simulink model "Longitudinal_Guide_130"  (Simulink 7.2)
settings: Solver=ode45  StartTime=0.0  StopTime=10.0  RelTol=1e-3
undefined symbols (not defined in the file or in its folder): DiscIntNeverNeededParam
libraries: simulink x1
settings Model: Creator=arnaud  LastModifiedBy=arnaud

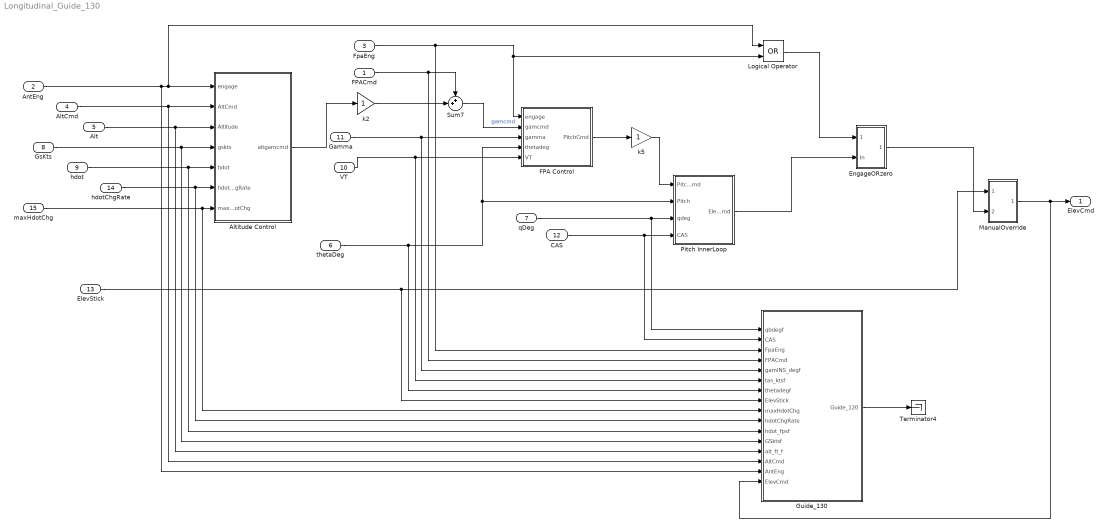
== system Longitudinal_Guide_130 ==
  FPACmd : Inport  DataType=double  OutDataTypeStr=double
  AntEng : Inport  Port=2  DataType=boolean  OutDataTypeStr=boolean
  FpaEng : Inport  Port=3  DataType=boolean  OutDataTypeStr=boolean
  AltCmd : Inport  Port=4  DataType=double  OutDataTypeStr=double
  Alt : Inport  Port=5  DataType=double  OutDataTypeStr=double
  thetaDeg : Inport  Port=6  DataType=double  OutDataTypeStr=double
  qDeg : Inport  Port=7  DataType=double  OutDataTypeStr=double
  GsKts : Inport  Port=8  DataType=double  OutDataTypeStr=double
  hdot : Inport  Port=9  DataType=double  OutDataTypeStr=double
  VT : Inport  Port=10  DataType=double  OutDataTypeStr=double
  Gamma : Inport  Port=11  DataType=double  OutDataTypeStr=double
  CAS : Inport  Port=12  DataType=double  OutDataTypeStr=double
  ElevStick : Inport  Port=13  DataType=double  OutDataTypeStr=double
  hdotChgRate : Inport  Port=14  DataType=double  OutDataTypeStr=double
  maxHdotChg : Inport  Port=15  DataType=double  OutDataTypeStr=double
  Altitude Control : Subsystem  RequirementInfo={'other' '..\..\tcm_requirements.docx' '@Simulink_requirement_item_14' 'true' 'Altitude Control' '' }  TreatAsAtomicUnit=on
  EngageORzero : Subsystem
  FPA Control : Subsystem  RequirementInfo={'other' '..\..\tcm_requirements.docx' '@Simulink_requirement_item_15' 'true' 'FPA Control' '' }  TreatAsAtomicUnit=on
  Guide_130 : Subsystem  TreatAsAtomicUnit=on  mask(Observer){AnnotationType=ensures, ObserverType=ellipsoid}
      mask prompts: AnnotationType "Type of annotation (pre/post...)"; ObserverType "Observer type"
      mask help:
      | Set an observer for the system.
      | The annotation type parameter sets the type of observer:
      | - requires : pre-condition
      | - ensures : post-condition
      | - assert : an assertion
      | - observer : the observer computes a special type of properties
      mask StyleString: popup(ensures|requires|assert|observer),edit
      mask CallbackString:
      | paramStr = get_param(gcb, 'MaskValues');
      | 
      | if strcmp(paramStr{1}(1),'o')
      |     set_param(gcb,'MaskVisibilities',{'on';'on'});
      |     paramStr{2} = 'ellipsoid';
      |     set_param(gcb,'MaskValues',paramStr);
      | else
      |     set_param(gcb,'MaskVisibilities',{'on';'off'});
      | end|paramStr = get_param(gcb, 'MaskValues');
      | 
      | if strcmp(paramStr{1}(1),'observer')
      |     set_param(gcb,'MaskVisibilities',{'on';'on'});
      |     paramStr{2} = 'ellipsoid';
      |     set_param(gcb,'MaskValues',paramStr);
      | else
      |     set_param(gcb,'MaskVisibilities',{'on';'off'});
      | end
      mask Display:
      | color('red');
      | text(0.5, 0.5, 'Observer Block', 'horizontalAlignment', 'center');
  Logical Operator : Logic  Operator=OR  AllPortsSameDT=off  OutDataTypeMode=boolean  OutDataTypeStr=boolean
  ManualOverride : Subsystem
  Pitch InnerLoop : Subsystem  RequirementInfo={'other' '..\..\tcm_requirements.docx' '@Simulink_requirement_item_17' 'true' 'Pitch InnerLoop' '' }  TreatAsAtomicUnit=on
  Sum7 : Sum  RequirementInfo={} %GIDa_92495686_3877_4412_b19f_22e099e095ee  Inputs=++|
  Terminator4 : Terminator
  k2 : Gain  RequirementInfo={} %GIDa_7e514706_5da4_4f1f_bf6c_0050dd9ce76d
  k5 : Gain  RequirementInfo={} %GIDa_b8b0ba7d_7fd3_4b03_b740_56530c3187c8
  ElevCmd : Outport
  wires:
  k2/1 -> Sum7/2
  Alt/1 -> Altitude Control/3(Altitude), Guide_130/13(alt_ft_f)
  thetaDeg/1 -> FPA Control/4(thetadeg), Pitch InnerLoop/2(Pitch), Guide_130/7(thetadegf)
  Gamma/1 -> FPA Control/3(gamma), Guide_130/5(gamINS_degf)
  AltCmd/1 -> Altitude Control/2(AltCmd), Guide_130/14(AltCmd)
  ManualOverride/1(Out) -> ElevCmd/1, Guide_130/16(ElevCmd)
  Altitude Control/1(altgamcmd) -> k2/1
  FPA Control/1(PitchCmd) -> k5/1
  hdot/1 -> Altitude Control/5(hdot), Guide_130/11(hdot_fpsf)
  Sum7/1 -> FPA Control/2(gamcmd)  "gamcmd"
  qDeg/1 -> Pitch InnerLoop/3(qdeg), Guide_130/1(qbdegf)
  GsKts/1 -> Altitude Control/4(gskts), Guide_130/12(GSktsf)
  VT/1 -> FPA Control/5(VT), Guide_130/6(tas_ktsf)
  FPACmd/1 -> Sum7/1, Guide_130/4(FPACmd)
  k5/1 -> Pitch InnerLoop/1(PitchCmd)
  FpaEng/1 -> Logical Operator/2, FPA Control/1(engage), Guide_130/3(FpaEng)
  CAS/1 -> Pitch InnerLoop/4(CAS), Guide_130/2(CAS)
  AntEng/1 -> Logical Operator/1, Altitude Control/1(engage), Guide_130/15(AntEng)
  ElevStick/1 -> ManualOverride/1(Man), Guide_130/8(ElevStick)
  Pitch InnerLoop/1(ElevCmd) -> EngageORzero/2(In)
  EngageORzero/1(Out) -> ManualOverride/2(Auto)
  Logical Operator/1 -> EngageORzero/1(Engage)
  maxHdotChg/1 -> Altitude Control/7(maxHdotChg), Guide_130/9(maxHdotChg)
  hdotChgRate/1 -> Altitude Control/6(hdotChgRate), Guide_130/10(hdotChgRate)
  Guide_130/1(Guide_120) -> Terminator4/1

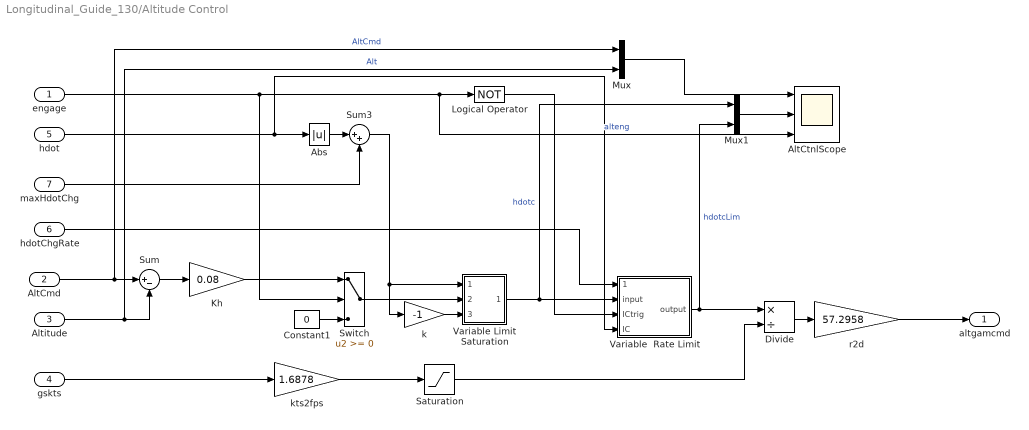
== system Longitudinal_Guide_130/Altitude Control ==
  engage : Inport  RequirementInfo={} %GIDa_92edc9e2_4cfd_4b16_8fee_8b94964575da
  AltCmd : Inport  RequirementInfo={} %GIDa_edbc7e5c_23e1_4d8f_98c5_e2d77895a510  Port=2
  Altitude : Inport  RequirementInfo={} %GIDa_01b40abf_ece8_4194_aeed_7639b2f9d320  Port=3
  gskts : Inport  RequirementInfo={} %GIDa_49aaf918_ec6b_4cc9_bdad_efb02f39ea3b  Port=4
  hdot : Inport  RequirementInfo={} %GIDa_f8353919_6ca2_40ed_9884_9c34b61b1365  Port=5
  hdotChgRate : Inport  Port=6
  maxHdotChg : Inport  Port=7
  Abs : Abs  RequirementInfo={} %GIDa_1391aa7c_5846_4be5_914e_111d8f2c4215  SaturateOnIntegerOverflow=on
  AltCtnlScope : Scope  NumInputPorts=3
      settings: RequirementInfo={} %GIDa_baad481c_a27b_41ac_bf32_d6e1a7f2cfe1  TimeRange=30  YMin=10000~-5~0  YMax=10200~15~1  SaveName=ScopeData3
  Constant1 : Constant  RequirementInfo={} %GIDa_566c4b52_316f_4d36_82bb_fb65e53f78d2  Value=0
  Divide : Product  RequirementInfo={} %GIDa_b9d1a3fe_7e00_46b2_9426_cf952dcaf391  Inputs=*/
  Kh : Gain  RequirementInfo={} %GIDa_de6b2d53_b3f4_42e2_83e9_439be9ccc299  Gain=0.08
  Logical Operator : Logic  RequirementInfo={} %GIDa_921e6188_0ac2_4a9c_befc_5c7a6835e9e6  Operator=NOT
  Mux : Mux  RequirementInfo={} %GIDa_68aa779e_2c07_4c3b_9ca1_0ecb3161e49a  Inputs=2
  Mux1 : Mux  RequirementInfo={} %GIDa_0a0909f8_d09a_4568_9828_3f29982a74b3  Inputs=2
  Saturation : Saturate  RequirementInfo={} %GIDa_77166b67_e163_40e1_b7e4_7e7410a56d29  UpperLimit=1000  LowerLimit=0.0001
  Sum : Sum  RequirementInfo={} %GIDa_d94a0856_9d8d_4fca_8b77_5f1cf21c0c3a  Inputs=|+-
  Sum3 : Sum  RequirementInfo={} %GIDa_3ee7802b_411f_4586_886f_8bdef6cfccb9  Inputs=|++  SaturateOnIntegerOverflow=on  InputSameDT=on  OutDataTypeStr=Inherit: Same as first input
  Switch : Switch  RequirementInfo={} %GIDa_64af29d5_be60_4de8_bcf5_833ab8e70f35
  Variable  Rate Limit : Subsystem  RequirementInfo={} %GIDa_7d0e1926_4469_4591_916e_2bb88ddee008  TreatAsAtomicUnit=on
  Variable Limit Saturation : Subsystem  RequirementInfo={} %GIDa_0b931211_59c1_4508_94b8_12d4cca2cb6b  TreatAsAtomicUnit=on
  k : Gain  RequirementInfo={} %GIDa_65a0c0b6_6e9b_4a97_b326_1d79079cc625  Gain=-1
  kts2fps : Gain  RequirementInfo={} %GIDa_a49848e7_9841_44de_8ec7_08f1ed28d1e0  Gain=1.6878
  r2d : Gain  RequirementInfo={} %GIDa_934ba914_aaac_471d_9b5e_a120031a3853  Gain=57.2958
  altgamcmd : Outport  RequirementInfo={} %GIDa_3c331913_004d_4e8f_a0a1_b052c80c7670
  wires:
  Sum/1 -> Kh/1
  AltCmd/1 -> Sum/1, Mux/1  "AltCmd"
  Altitude/1 -> Sum/2, Mux/2  "Alt"
  hdot/1 -> Abs/1, Variable  Rate Limit/4(IC)
  Abs/1 -> Sum3/1
  maxHdotChg/1 -> Sum3/2
  k/1 -> Variable Limit Saturation/3(Lo_lim)
  Sum3/1 -> k/1, Variable Limit Saturation/1(up_lim)
  engage/1 -> Switch/2, Logical Operator/1, AltCtnlScope/3  "alteng"
  gskts/1 -> kts2fps/1
  Divide/1 -> r2d/1
  r2d/1 -> altgamcmd/1
  Logical Operator/1 -> Variable  Rate Limit/3(ICtrig)
  Variable Limit Saturation/1(Out1) -> Variable  Rate Limit/2(input), Mux1/1  "hdotc"
  hdotChgRate/1 -> Variable  Rate Limit/1(ratelim)
  Variable  Rate Limit/1(output) -> Divide/1, Mux1/2  "hdotcLim"
  kts2fps/1 -> Saturation/1
  Saturation/1 -> Divide/2
  Switch/1 -> Variable Limit Saturation/2(SigIn)
  Kh/1 -> Switch/1
  Constant1/1 -> Switch/3
  Mux/1 -> AltCtnlScope/1
  Mux1/1 -> AltCtnlScope/2

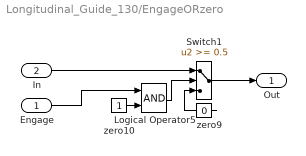
== system Longitudinal_Guide_130/EngageORzero ==
  Engage : Inport
  In : Inport  Port=2
  Logical Operator5 : Logic  RequirementInfo={} %GIDa_2faaa958_fdd5_4161_8224_87bc655595ec  AllPortsSameDT=off  OutDataTypeMode=boolean  OutDataTypeStr=boolean
  Switch1 : Switch  RequirementInfo={} %GIDa_cd8505b1_f38c_41a3_a83c_5e083797b181  Threshold=0.5
  zero10 : Constant  RequirementInfo={} %GIDa_596a5899_ba53_4c37_8272_7211e27ddf24
  zero9 : Constant  RequirementInfo={} %GIDa_b5c8c028_3d9d_45c0_afd9_41cf87627ef7  Value=0
  Out : Outport
  wires:
  Engage/1 -> Logical Operator5/1
  zero10/1 -> Logical Operator5/2
  zero9/1 -> Switch1/3
  In/1 -> Switch1/1
  Logical Operator5/1 -> Switch1/2
  Switch1/1 -> Out/1

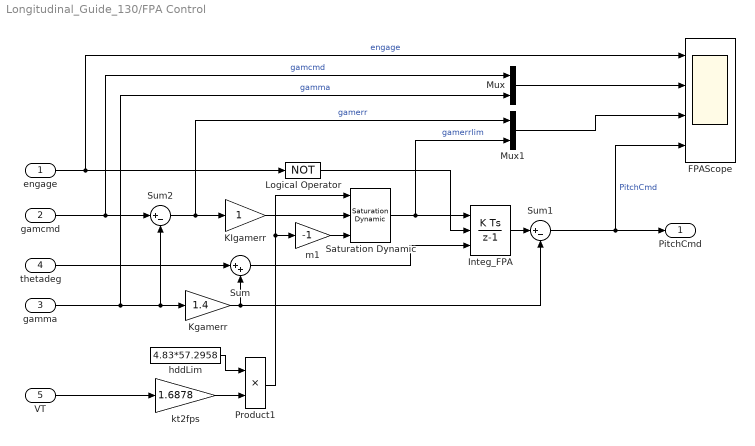
== system Longitudinal_Guide_130/FPA Control ==
  engage : Inport  RequirementInfo={} %GIDa_4330a6b4_8fd7_4be4_8132_0a5a51cb5321
  gamcmd : Inport  RequirementInfo={} %GIDa_72bd14a4_cf4e_4ddf_9979_bc189fd4e864  Port=2
  gamma : Inport  RequirementInfo={} %GIDa_07a290a4_e9be_4e9c_ae2b_d72f5ca4cb2b  Port=3
  thetadeg : Inport  RequirementInfo={} %GIDa_6ddd8d11_1197_4928_a2bc_231a82446ee7  Port=4
  VT : Inport  RequirementInfo={} %GIDa_a0a43ff9_fad6_4fc8_a8cd_c357b3dfb673  Port=5
  FPAScope : Scope  NumInputPorts=4
      settings: RequirementInfo={} %GIDa_08c55925_5efe_4d90_b09d_0072cafa98d7  YMin=-1~-5~-2~-5  YMax=2~5~2~10  SaveName=ScopeData12
  Integ_FPA : DiscreteIntegrator  ExternalReset=level  InitialConditionSource=external  SampleTime=1.0  ICPrevOutput=DiscIntNeverNeededParam  ICPrevScaledInput=DiscIntNeverNeededParam  mask(DiscretizedDiscreteIntegrator){}
      mask init:
      | %zoh
  KIgamerr : Gain  RequirementInfo={} %GIDa_08963e9e_c311_47c8_a63e_11cc7c9fb2d8
  Kgamerr : Gain  RequirementInfo={} %GIDa_3495b1a6_277d_4a6c_aa4f_649fc83b9092  Gain=1.4
  Logical Operator : Logic  RequirementInfo={} %GIDa_eba75fd0_479d_4894_b4e0_0ecea241815c  Operator=NOT  AllPortsSameDT=off  OutDataTypeMode=boolean  OutDataTypeStr=boolean
  Mux : Mux  RequirementInfo={} %GIDa_ae1e9d70_29ff_4004_97f5_396f2626ff0e  Inputs=2
  Mux1 : Mux  RequirementInfo={} %GIDa_b657458f_9c9c_48b1_af95_f550cfeae5f6  Inputs=2
  Product1 : Product  RequirementInfo={} %GIDa_bb863780_5e58_4e21_8791_e7a2c94dd786  RndMeth=Zero
  Saturation Dynamic : simulink/Discontinuities/Saturation Dynamic  SystemSampleTime=-1  OutMin=[]  OutMax=[]  OutDataTypeStr=Inherit: Same as second input  OutDataType=fixdt(1, 16)  OutScaling=2^-10  DoSatur=off
  Sum : Sum  RequirementInfo={} %GIDa_494c7255_4427_4dad_a3c1_4aee399936eb  Inputs=|++
  Sum1 : Sum  RequirementInfo={} %GIDa_93359946_60e9_438e_99e8_9beddee58b77  Inputs=|+-
  Sum2 : Sum  RequirementInfo={} %GIDa_c5e9feb7_f19d_4066_9b64_2fe045a465c2  Inputs=|+-
  hddLim : Constant  RequirementInfo={} %GIDa_1bf124ef_f3a0_4770_a704_52ef6436d4b5  Value=4.83*57.2958
  kt2fps : Gain  RequirementInfo={} %GIDa_c7ee5a6f_140d_48a3_b5c5_8ced7bef0603  Gain=1.6878
  m1 : Gain  RequirementInfo={} %GIDa_3e310fb8_58d1_4ad2_a1bc_b1914379a108  Gain=-1
  PitchCmd : Outport  RequirementInfo={} %GIDa_7e56bb7b_bd21_4466_8889_6a6d9858a2da
  wires:
  Sum1/1 -> PitchCmd/1, FPAScope/4  "PitchCmd"
  Kgamerr/1 -> Sum1/2, Sum/2
  Integ_FPA/1 -> Sum1/1
  gamma/1 -> Kgamerr/1, Sum2/2, Mux/2  "gamma"
  thetadeg/1 -> Sum/1
  Sum/1 -> Integ_FPA/3
  engage/1 -> Logical Operator/1, FPAScope/1  "engage"
  Logical Operator/1 -> Integ_FPA/2
  kt2fps/1 -> Product1/2
  hddLim/1 -> Product1/1
  Product1/1 -> Saturation Dynamic/1, m1/1
  VT/1 -> kt2fps/1
  Saturation Dynamic/1 -> Integ_FPA/1, Mux1/2  "gamerrlim"
  KIgamerr/1 -> Saturation Dynamic/2
  m1/1 -> Saturation Dynamic/3
  Sum2/1 -> KIgamerr/1, Mux1/1  "gamerr"
  gamcmd/1 -> Sum2/1, Mux/1  "gamcmd"
  Mux/1 -> FPAScope/2
  Mux1/1 -> FPAScope/3

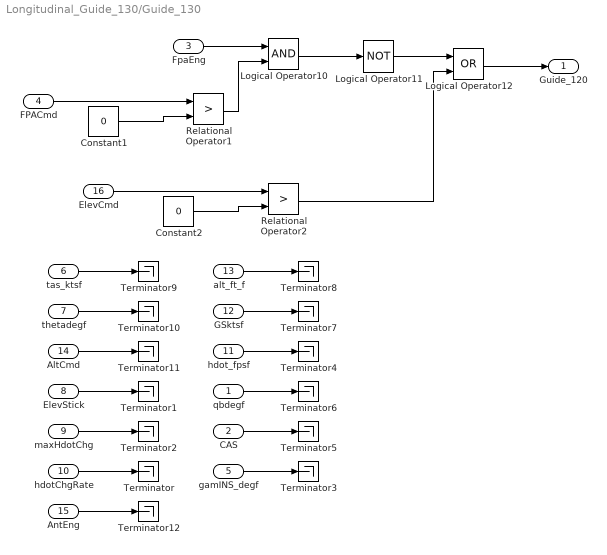
== system Longitudinal_Guide_130/Guide_130 ==
  qbdegf : Inport  OutDataType=sfix(16)  OutScaling=2^0
  CAS : Inport  Port=2  OutDataType=sfix(16)  OutScaling=2^0
  FpaEng : Inport  Port=3  OutDataType=sfix(16)  OutScaling=2^0
  FPACmd : Inport  Port=4  OutDataType=sfix(16)  OutScaling=2^0
  gamINS_degf : Inport  Port=5  OutDataType=sfix(16)  OutScaling=2^0
  tas_ktsf : Inport  Port=6  OutDataType=sfix(16)  OutScaling=2^0
  thetadegf : Inport  Port=7  OutDataType=sfix(16)  OutScaling=2^0
  ElevStick : Inport  Port=8  OutDataType=sfix(16)  OutScaling=2^0
  maxHdotChg : Inport  Port=9  OutDataType=sfix(16)  OutScaling=2^0
  hdotChgRate : Inport  Port=10  OutDataType=sfix(16)  OutScaling=2^0
  hdot_fpsf : Inport  Port=11  OutDataType=sfix(16)  OutScaling=2^0
  GSktsf : Inport  Port=12  OutDataType=sfix(16)  OutScaling=2^0
  alt_ft_f : Inport  Port=13  OutDataType=sfix(16)  OutScaling=2^0
  AltCmd : Inport  Port=14  OutDataType=sfix(16)  OutScaling=2^0
  AntEng : Inport  Port=15  OutDataType=sfix(16)  OutScaling=2^0
  ElevCmd : Inport  Port=16  OutDataType=sfix(16)  OutScaling=2^0
  Constant1 : Constant  Value=0  OutDataType=sfix(16)  OutScaling=2^0
  Constant2 : Constant  Value=0  OutDataType=sfix(16)  OutScaling=2^0
  Logical Operator10 : Logic  AllPortsSameDT=off  OutDataTypeMode=boolean  OutDataTypeStr=boolean
  Logical Operator11 : Logic  Operator=NOT  AllPortsSameDT=off  OutDataTypeMode=boolean  OutDataTypeStr=boolean
  Logical Operator12 : Logic  Operator=OR  AllPortsSameDT=off  OutDataTypeMode=boolean  OutDataTypeStr=boolean
  Relational Operator1 : RelationalOperator  Operator=>  LogicOutDataTypeMode=boolean  OutDataTypeStr=boolean
  Relational Operator2 : RelationalOperator  Operator=>  LogicOutDataTypeMode=boolean  OutDataTypeStr=boolean
  Terminator{,1..12} (13 alike) : Terminator
  Guide_120 : Outport  OutDataType=sfix(16)  OutScaling=2^0
  wires:
  hdotChgRate/1 -> Terminator/1
  maxHdotChg/1 -> Terminator2/1
  ElevStick/1 -> Terminator1/1
  CAS/1 -> Terminator5/1
  qbdegf/1 -> Terminator6/1
  Constant2/1 -> Relational Operator2/2
  ElevCmd/1 -> Relational Operator2/1
  FpaEng/1 -> Logical Operator10/1
  Constant1/1 -> Relational Operator1/2
  FPACmd/1 -> Relational Operator1/1
  Relational Operator1/1 -> Logical Operator10/2
  Logical Operator11/1 -> Logical Operator12/1
  Logical Operator10/1 -> Logical Operator11/1
  Relational Operator2/1 -> Logical Operator12/2
  Logical Operator12/1 -> Guide_120/1
  alt_ft_f/1 -> Terminator8/1
  GSktsf/1 -> Terminator7/1
  hdot_fpsf/1 -> Terminator4/1
  gamINS_degf/1 -> Terminator3/1
  tas_ktsf/1 -> Terminator9/1
  thetadegf/1 -> Terminator10/1
  AltCmd/1 -> Terminator11/1
  AntEng/1 -> Terminator12/1

== system Longitudinal_Guide_130/ManualOverride ==
  Man : Inport
  Auto : Inport  Port=2
  Switch1 : Switch  RequirementInfo={} %GIDa_891c72b6_c029_43c0_848a_219761f8f015  Criteria=u2 ~= 0  Threshold=0.5
  Out : Outport
  wires:
  Man/1 -> Switch1/3, Switch1/2
  Auto/1 -> Switch1/1
  Switch1/1 -> Out/1

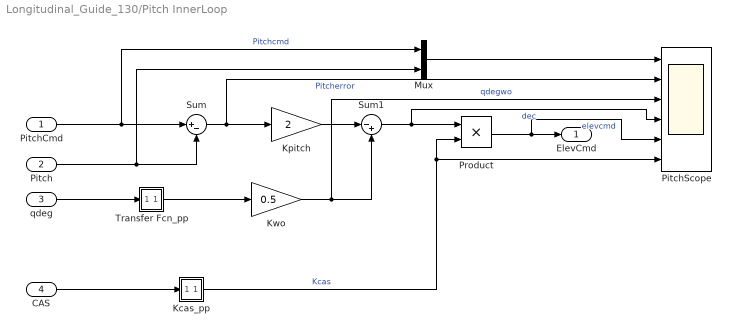
== system Longitudinal_Guide_130/Pitch InnerLoop ==
  PitchCmd : Inport  RequirementInfo={} %GIDa_e681796d_a620_4c95_b4ed_ba3232dc70a2
  Pitch : Inport  RequirementInfo={} %GIDa_6f4baf24_a090_49e6_89b2_2ff3bd4fd377  Port=2
  qdeg : Inport  RequirementInfo={} %GIDa_13210493_e26c_4a14_89fc_8ad0299ca616  Port=3
  CAS : Inport  RequirementInfo={} %GIDa_e1a07f62_5dbf_46dc_bc2c_c2998ea01de8  Port=4
  Kcas_pp : Subsystem  TreatAsAtomicUnit=on
  Kpitch : Gain  RequirementInfo={} %GIDa_4a392bdb_3184_422c_b598_a156d3e8b02c  Gain=2
  Kwo : Gain  RequirementInfo={} %GIDa_6174b3c5_b132_42d6_a380_7a86f841c8e6  Gain=0.5
  Mux : Mux  RequirementInfo={} %GIDa_93279ee0_cc4a_4a25_b0b1_b731353743b0  Inputs=2
  PitchScope : Scope  NumInputPorts=6
      settings: RequirementInfo={} %GIDa_5646223d_16bd_44bf_9f51_c97977b5f9c0  YMin=-2~-2~-2~-20~-20~0  YMax=10~2~2~20~20~1.2  SaveName=ScopeData11
  Product : Product  RequirementInfo={} %GIDa_ee2099f1_df06_4fc6_bf9b_0b7652de3a20  RndMeth=Zero
  Sum : Sum  RequirementInfo={} %GIDa_6e966264_2a04_4ed3_91bc_90c4039fd9a0  Inputs=|+-
  Sum1 : Sum  RequirementInfo={} %GIDa_5254d09e_07d7_42ec_bb70_93117997e359  Inputs=|-+
  Transfer Fcn_pp : Subsystem  TreatAsAtomicUnit=on
  ElevCmd : Outport  RequirementInfo={} %GIDa_133d9978_a863_4cc3_b149_7ebb5beb5068
  wires:
  Sum/1 -> Kpitch/1, PitchScope/2  "Pitcherror"
  Pitch/1 -> Sum/2, Mux/2
  Kpitch/1 -> Sum1/1
  qdeg/1 -> Transfer Fcn_pp/1(Inport1)
  Transfer Fcn_pp/1(Outport1) -> Kwo/1
  CAS/1 -> Kcas_pp/1(In)
  Sum1/1 -> Product/1, PitchScope/4  "dec"
  Kcas_pp/1(Out) -> Product/2, PitchScope/6  "Kcas"
  Product/1 -> ElevCmd/1, PitchScope/5  "elevcmd"
  Kwo/1 -> Sum1/2, PitchScope/3  "qdegwo"
  PitchCmd/1 -> Sum/1, Mux/1  "Pitchcmd"
  Mux/1 -> PitchScope/1

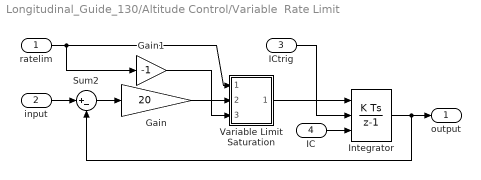
== system Longitudinal_Guide_130/Altitude Control/Variable  Rate Limit ==
  ratelim : Inport  RequirementInfo={} %GIDa_1ef85aab_f902_404e_a68b_00e57673dd3f
  input : Inport  RequirementInfo={} %GIDa_7ac59940_1fcc_4039_a5aa_a007950c590e  Port=2
  ICtrig : Inport  RequirementInfo={} %GIDa_9850dee7_08ca_49d5_88fb_399ee4ba203e  Port=3
  IC : Inport  RequirementInfo={} %GIDa_d80fe626_91fd_4f82_ad17_86aca6b3aee5  Port=4
  Gain : Gain  RequirementInfo={} %GIDa_55467e41_3bd6_44bf_9a44_6f78661bf8f0  Gain=20  SaturateOnIntegerOverflow=on  OutDataTypeStr=Inherit: Same as input  ParamDataTypeStr=Inherit: Same as input
  Gain1 : Gain  RequirementInfo={} %GIDa_0b7dd2e9_dfcf_42d3_8fb1_8c254e005ceb  Gain=-1  SaturateOnIntegerOverflow=on  OutDataTypeStr=Inherit: Same as input  ParamDataTypeStr=Inherit: Same as input
  Integrator : DiscreteIntegrator  ExternalReset=level  InitialConditionSource=external  SampleTime=1.0  ICPrevOutput=DiscIntNeverNeededParam  ICPrevScaledInput=DiscIntNeverNeededParam  mask(DiscretizedDiscreteIntegrator){}
      mask init:
      | %zoh
  Sum2 : Sum  RequirementInfo={} %GIDa_de9ff84b_54f5_48bc_9ef3_874415208380  Inputs=|+-  SaturateOnIntegerOverflow=on
  Variable Limit Saturation : Subsystem  RequirementInfo={} %GIDa_42540829_63e9_4d83_adf5_d7c684208c2d
  output : Outport  RequirementInfo={} %GIDa_74eb2916_410f_4b2d_afdf_0d476e7e03b7
  wires:
  Sum2/1 -> Gain/1
  Gain/1 -> Variable Limit Saturation/2(SigIn)
  ratelim/1 -> Gain1/1, Variable Limit Saturation/1(up_lim)
  Gain1/1 -> Variable Limit Saturation/3(Lo_lim)
  Variable Limit Saturation/1(Out1) -> Integrator/1
  Integrator/1 -> Sum2/2, output/1
  input/1 -> Sum2/1
  ICtrig/1 -> Integrator/2
  IC/1 -> Integrator/3

== system Longitudinal_Guide_130/Altitude Control/Variable Limit Saturation ==
  up_lim : Inport  RequirementInfo={} %GIDa_a8c5a358_1294_4ae6_a63f_3940fe218386
  SigIn : Inport  RequirementInfo={} %GIDa_062a0af8_40f0_4204_856b_8e0aded8de05  Port=2
  Lo_lim : Inport  RequirementInfo={} %GIDa_6793747b_c094_4bd9_a5cb_839f8eb54e21  Port=3
  Enforce low lim : MinMax  RequirementInfo={} %GIDa_e93f4b97_2f8b_4f52_84c9_3cb68ddf7e16  Function=max  Inputs=2
  Enforce up lim : MinMax  RequirementInfo={} %GIDa_c018e6ad_c664_4361_a96c_d990e2efb7d8  Inputs=2
  Out1 : Outport  RequirementInfo={} %GIDa_0d7a9d35_dde5_41a4_a708_f2de214bfa54
  wires:
  Lo_lim/1 -> Enforce low lim/1
  SigIn/1 -> Enforce low lim/2
  Enforce low lim/1 -> Enforce up lim/1
  up_lim/1 -> Enforce up lim/2
  Enforce up lim/1 -> Out1/1

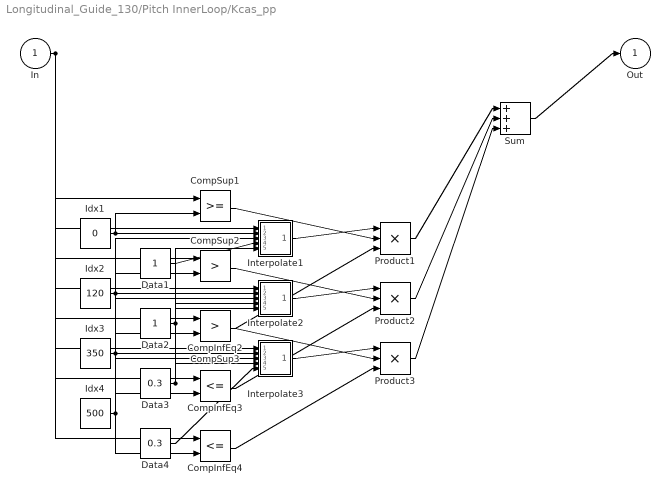
== system Longitudinal_Guide_130/Pitch InnerLoop/Kcas_pp ==
  In : Inport
  CompInfEq2 : RelationalOperator  Operator=<=  InputSameDT=on
  CompInfEq3 : RelationalOperator  Operator=<=  InputSameDT=on
  CompInfEq4 : RelationalOperator  Operator=<=  InputSameDT=on
  CompSup1 : RelationalOperator  InputSameDT=on
  CompSup2 : RelationalOperator  Operator=>  InputSameDT=on
  CompSup3 : RelationalOperator  Operator=>  InputSameDT=on
  Data1 : Constant
  Data2 : Constant
  Data3 : Constant  Value=0.3
  Data4 : Constant  Value=0.3
  Idx1 : Constant  Value=0
  Idx2 : Constant  Value=120
  Idx3 : Constant  Value=350
  Idx4 : Constant  Value=500
  Interpolate1 : Subsystem
  Interpolate2 : Subsystem
  Interpolate3 : Subsystem
  Product1 : Product  Inputs=***  SaturateOnIntegerOverflow=on  RndMeth=Zero  OutDataTypeStr=Inherit: Same as first input
  Product2 : Product  Inputs=***  SaturateOnIntegerOverflow=on  RndMeth=Zero  OutDataTypeStr=Inherit: Same as first input
  Product3 : Product  Inputs=***  SaturateOnIntegerOverflow=on  RndMeth=Zero  OutDataTypeStr=Inherit: Same as first input
  Sum : Sum  Inputs=+++  SaturateOnIntegerOverflow=on  InputSameDT=on  OutDataTypeStr=Inherit: Same as first input
  Out : Outport
  wires:
  In/1 -> Interpolate1/1(InportIn), CompSup1/1, Interpolate2/1(InportIn), CompSup2/1, CompInfEq2/1, Interpolate3/1(InportIn), CompSup3/1, CompInfEq3/1, CompInfEq4/1
  Idx1/1 -> Interpolate1/2(InportIdx1), CompSup1/2
  Data1/1 -> Interpolate1/4(InportData1)
  Interpolate1/1(Out) -> Product1/1
  CompSup1/1 -> Product1/2
  CompInfEq2/1 -> Product1/3
  Product1/1 -> Sum/1
  Idx2/1 -> Interpolate2/2(InportIdx1), CompSup2/2, Interpolate1/3(InportIdx2), CompInfEq2/2
  Data2/1 -> Interpolate2/4(InportData1), Interpolate1/5(InportData2)
  Interpolate2/1(Out) -> Product2/1
  CompSup2/1 -> Product2/2
  CompInfEq3/1 -> Product2/3
  Product2/1 -> Sum/2
  Idx3/1 -> Interpolate3/2(InportIdx1), CompSup3/2, Interpolate2/3(InportIdx2), CompInfEq3/2
  Data3/1 -> Interpolate3/4(InportData1), Interpolate2/5(InportData2)
  Interpolate3/1(Out) -> Product3/1
  CompSup3/1 -> Product3/2
  CompInfEq4/1 -> Product3/3
  Product3/1 -> Sum/3
  Idx4/1 -> Interpolate3/3(InportIdx2), CompInfEq4/2
  Data4/1 -> Interpolate3/5(InportData2)
  Sum/1 -> Out/1

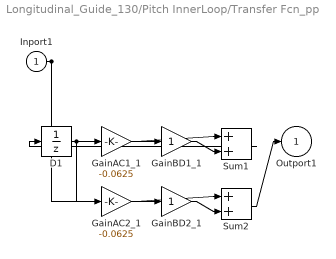
== system Longitudinal_Guide_130/Pitch InnerLoop/Transfer Fcn_pp ==
  Inport1 : Inport
  D1 : UnitDelay  SampleTime=-1
  GainAC1_1 : Gain  Gain=-0.0625  SaturateOnIntegerOverflow=on  OutDataTypeStr=Inherit: Same as input  ParamDataTypeStr=Inherit: Same as input
  GainAC2_1 : Gain  Gain=-0.0625  SaturateOnIntegerOverflow=on  OutDataTypeStr=Inherit: Same as input  ParamDataTypeStr=Inherit: Same as input
  GainBD1_1 : Gain  SaturateOnIntegerOverflow=on  OutDataTypeStr=Inherit: Same as input  ParamDataTypeStr=Inherit: Same as input
  GainBD2_1 : Gain  SaturateOnIntegerOverflow=on  OutDataTypeStr=Inherit: Same as input  ParamDataTypeStr=Inherit: Same as input
  Sum1 : Sum  SaturateOnIntegerOverflow=on  InputSameDT=on  OutDataTypeStr=Inherit: Same as first input
  Sum2 : Sum  SaturateOnIntegerOverflow=on  InputSameDT=on  OutDataTypeStr=Inherit: Same as first input
  Outport1 : Outport
  wires:
  D1/1 -> GainAC1_1/1, GainAC2_1/1
  GainAC1_1/1 -> Sum1/1
  GainAC2_1/1 -> Sum2/1
  Inport1/1 -> GainBD1_1/1, GainBD2_1/1
  GainBD1_1/1 -> Sum1/2
  GainBD2_1/1 -> Sum2/2
  Sum1/1 -> D1/1
  Sum2/1 -> Outport1/1

== system Longitudinal_Guide_130/Altitude Control/Variable  Rate Limit/Variable Limit Saturation ==
  up_lim : Inport  RequirementInfo={} %GIDa_c3426702_ae57_4a6b_8e5b_d8e7ea7997b8
  SigIn : Inport  RequirementInfo={} %GIDa_57ffe4bd_514b_4f1d_925b_ea07d6710330  Port=2
  Lo_lim : Inport  RequirementInfo={} %GIDa_934c3ebb_c2a8_4cb2_b1d4_7a7b38287908  Port=3
  Enforce low lim : MinMax  RequirementInfo={} %GIDa_f320f771_b833_4e25_ab12_e91693dd9b04  Function=max  Inputs=2
  Enforce up lim : MinMax  RequirementInfo={} %GIDa_1cfdde9a_faa1_4e7e_9516_cacb3f0cb773  Inputs=2
  Out1 : Outport  RequirementInfo={} %GIDa_6b324e36_3b21_43eb_ae92_bdd39356922a
  wires:
  Enforce up lim/1 -> Out1/1
  up_lim/1 -> Enforce up lim/2
  Enforce low lim/1 -> Enforce up lim/1
  SigIn/1 -> Enforce low lim/2
  Lo_lim/1 -> Enforce low lim/1

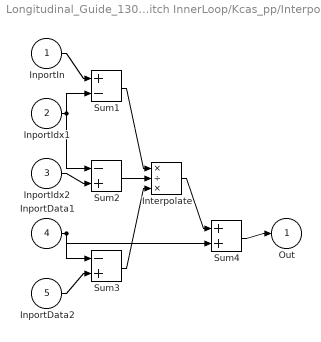
== system Longitudinal_Guide_130/Pitch InnerLoop/Kcas_pp/Interpolate1 ==
  InportIn : Inport
  InportIdx1 : Inport  Port=2
  InportIdx2 : Inport  Port=3
  InportData1 : Inport  Port=4
  InportData2 : Inport  Port=5
  Interpolate : Product  Inputs=*/*  SaturateOnIntegerOverflow=on  RndMeth=Zero  InputSameDT=on  OutDataTypeStr=Inherit: Same as first input
  Sum1 : Sum  Inputs=+-  SaturateOnIntegerOverflow=on  InputSameDT=on  OutDataTypeStr=Inherit: Same as first input
  Sum2 : Sum  Inputs=-+  SaturateOnIntegerOverflow=on  InputSameDT=on  OutDataTypeStr=Inherit: Same as first input
  Sum3 : Sum  Inputs=-+  SaturateOnIntegerOverflow=on  InputSameDT=on  OutDataTypeStr=Inherit: Same as first input
  Sum4 : Sum  SaturateOnIntegerOverflow=on  InputSameDT=on  OutDataTypeStr=Inherit: Same as first input
  Out : Outport
  wires:
  InportIn/1 -> Sum1/1
  InportIdx1/1 -> Sum1/2, Sum2/1
  InportIdx2/1 -> Sum2/2
  InportData1/1 -> Sum3/1, Sum4/2
  InportData2/1 -> Sum3/2
  Sum1/1 -> Interpolate/1
  Sum2/1 -> Interpolate/2
  Sum3/1 -> Interpolate/3
  Interpolate/1 -> Sum4/1
  Sum4/1 -> Out/1

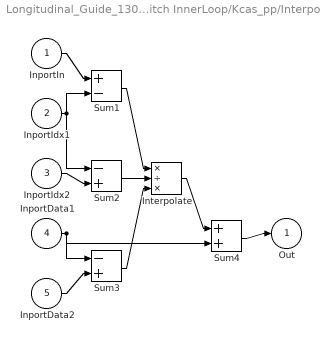
== system Longitudinal_Guide_130/Pitch InnerLoop/Kcas_pp/Interpolate2 ==
  InportIn : Inport
  InportIdx1 : Inport  Port=2
  InportIdx2 : Inport  Port=3
  InportData1 : Inport  Port=4
  InportData2 : Inport  Port=5
  Interpolate : Product  Inputs=*/*  SaturateOnIntegerOverflow=on  RndMeth=Zero  InputSameDT=on  OutDataTypeStr=Inherit: Same as first input
  Sum1 : Sum  Inputs=+-  SaturateOnIntegerOverflow=on  InputSameDT=on  OutDataTypeStr=Inherit: Same as first input
  Sum2 : Sum  Inputs=-+  SaturateOnIntegerOverflow=on  InputSameDT=on  OutDataTypeStr=Inherit: Same as first input
  Sum3 : Sum  Inputs=-+  SaturateOnIntegerOverflow=on  InputSameDT=on  OutDataTypeStr=Inherit: Same as first input
  Sum4 : Sum  SaturateOnIntegerOverflow=on  InputSameDT=on  OutDataTypeStr=Inherit: Same as first input
  Out : Outport
  wires:
  InportIn/1 -> Sum1/1
  InportIdx1/1 -> Sum1/2, Sum2/1
  InportIdx2/1 -> Sum2/2
  InportData1/1 -> Sum3/1, Sum4/2
  InportData2/1 -> Sum3/2
  Sum1/1 -> Interpolate/1
  Sum2/1 -> Interpolate/2
  Sum3/1 -> Interpolate/3
  Interpolate/1 -> Sum4/1
  Sum4/1 -> Out/1

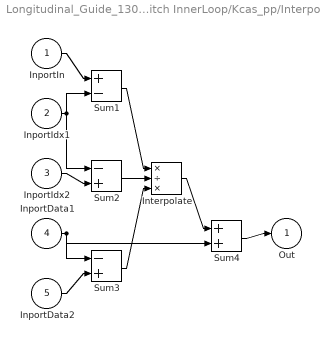
== system Longitudinal_Guide_130/Pitch InnerLoop/Kcas_pp/Interpolate3 ==
  InportIn : Inport
  InportIdx1 : Inport  Port=2
  InportIdx2 : Inport  Port=3
  InportData1 : Inport  Port=4
  InportData2 : Inport  Port=5
  Interpolate : Product  Inputs=*/*  SaturateOnIntegerOverflow=on  RndMeth=Zero  InputSameDT=on  OutDataTypeStr=Inherit: Same as first input
  Sum1 : Sum  Inputs=+-  SaturateOnIntegerOverflow=on  InputSameDT=on  OutDataTypeStr=Inherit: Same as first input
  Sum2 : Sum  Inputs=-+  SaturateOnIntegerOverflow=on  InputSameDT=on  OutDataTypeStr=Inherit: Same as first input
  Sum3 : Sum  Inputs=-+  SaturateOnIntegerOverflow=on  InputSameDT=on  OutDataTypeStr=Inherit: Same as first input
  Sum4 : Sum  SaturateOnIntegerOverflow=on  InputSameDT=on  OutDataTypeStr=Inherit: Same as first input
  Out : Outport
  wires:
  InportIn/1 -> Sum1/1
  InportIdx1/1 -> Sum1/2, Sum2/1
  InportIdx2/1 -> Sum2/2
  InportData1/1 -> Sum3/1, Sum4/2
  InportData2/1 -> Sum3/2
  Sum1/1 -> Interpolate/1
  Sum2/1 -> Interpolate/2
  Sum3/1 -> Interpolate/3
  Interpolate/1 -> Sum4/1
  Sum4/1 -> Out/1
